simulink model "counter"  (R2012b)
settings: Solver=ode45  StartTime=0.0  StopTime=10.0  RelTol=1e-3
settings Model: Creator=MSuP  LastModifiedBy=MSuP
settings OptimizationCC: InlineParams=on

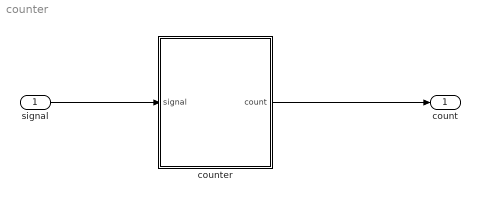
== system counter ==
  "signal " : Inport
  counter : Stateflow chart  TreatAsAtomicUnit=on
  count : Outport
  wires:
  "signal "/1 -> counter/1(signal)
  counter/1(count) -> count/1

== stateflow chart counter/counter ==
  state counter
    en:lastSignal=signal;
    count = internalCounter;
  (default) -> counter
  (junction 7) -> counter [order 2]
  counter -> (junction 7) : [signal != lastSignal]
  (junction 7) -> counter [order 1] : [signal > lastSignal] {internalCounter += 1}
  data: signal input; count output double; lastSignal local double; internalCounter local double =0
